simulink model "SL_Practica_3"  (R2024a)
settings: Solver=VariableStepAuto  StartTime=0.0  StopTime=20  RelTol=1e-3
values from neighbouring files (symbols this model uses):
  b1 = 1000    [Parametros_SL_P3.m]    (also in Practica_3.m)
  k1 = 16182    [Parametros_SL_P3.m]    (also in Practica_3.m)
  k2 = 19000    [Parametros_SL_P3.m]    (also in Practica_3.m)
  m1 = 290    [Parametros_SL_P3.m]    (also in Practica_3.m)
  m2 = 59    [Parametros_SL_P3.m]    (also in Practica_3.m)

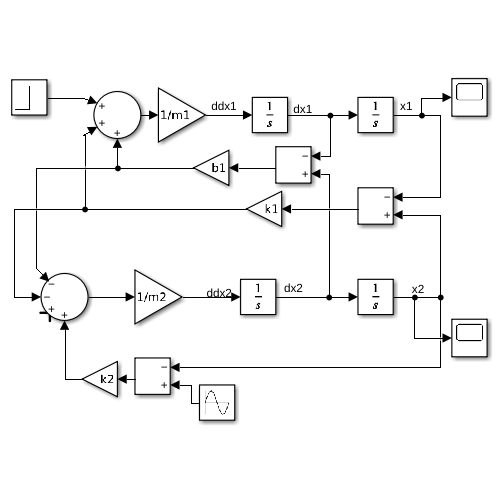
[thumbnail: Simulink's stored preview of the top-level diagram]
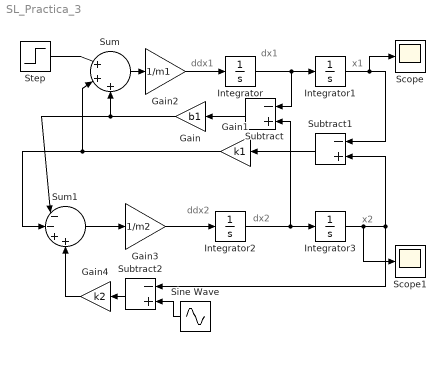
== system SL_Practica_3 ==
  note: x2
  note: dx2
  note: ddx2
  note: x1
  note: dx1
  note: ddx1
  Gain : Gain  Gain=b1
  Gain1 : Gain  Gain=k1
  Gain2 : Gain  Gain=1/m1
  Gain3 : Gain  Gain=1/m2
  Gain4 : Gain  Gain=k2
  Integrator{,1..3} (4 alike) : Integrator
  Scope : Scope
  Scope1 : Scope
  Sine Wave : Sin  Amplitude=0.05  Frequency=0.5*pi  SampleTime=0
  Step : Step  Time=0  After=0  SampleTime=0
  Subtract : Sum  Inputs=-+
  Subtract1 : Sum  Inputs=-+
  Subtract2 : Sum  Inputs=-+
  Sum : Sum  Inputs=|+++
  Sum1 : Sum  Inputs=|--++
  wires:
  Integrator/1 -> Subtract/1, Integrator1/1
  Gain2/1 -> Integrator/1
  Subtract/1 -> Gain/1
  Subtract1/1 -> Gain1/1
  Integrator1/1 -> Scope/1, Subtract1/1
  Gain/1 -> Sum1/1, Sum/3
  Gain1/1 -> Sum1/2, Sum/2
  Sum/1 -> Gain2/1
  Gain3/1 -> Integrator2/1
  Integrator2/1 -> Subtract/2, Integrator3/1
  Sine Wave/1 -> Subtract2/2
  Integrator3/1 -> Scope1/1, Subtract2/1, Subtract1/2
  Subtract2/1 -> Gain4/1
  Sum1/1 -> Gain3/1
  Gain4/1 -> Sum1/4
  Step/1 -> Sum/1
